simulink model "updatedoldEMS_Gyro_Model"  (R2024a)
settings: Solver=FixedStepAuto  StartTime=0.0  StopTime=360  FixedStep=1/16  RelTol=1e-3
libraries: simulink x1, aerolibnav x1
settings Model: Creator=stevalmontxy  LastModifiedBy=sxyan
settings RTWCC: GPUComputeCapability=3.5

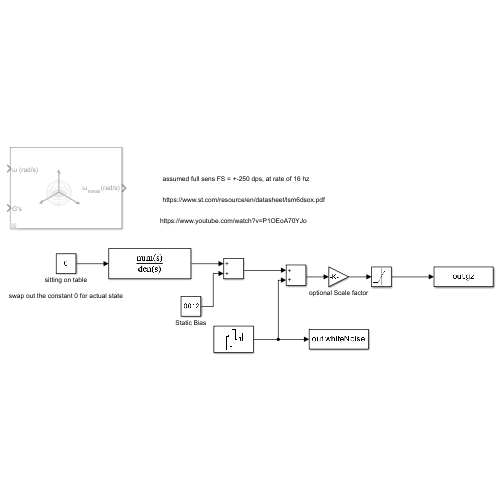
[thumbnail: Simulink's stored preview of the top-level diagram]
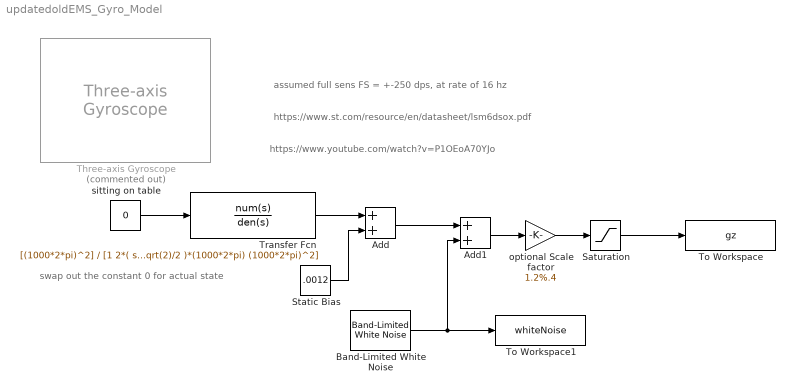
== system updatedoldEMS_Gyro_Model ==
  note: swap out the constant 0 for actual state
  note: https://www.st.com/resource/en/datasheet/lsm6dsox.pdf
  note: assumed full sens FS = +-250 dps, at rate of 16 hz
  note: https://www.youtube.com/watch?v=P1OEoA70YJo
  Add : Sum
  Add1 : Sum
  Band-Limited White Noise : simulink/Sources/Band-Limited White Noise  Cov=".004443^2 %  .0038^2 %"  Ts=1/16  seed=[23341]
  Saturation : Saturate  UpperLimit=2^15  LowerLimit=-2^15
  Static Bias : Constant  Value=.0012
  Three-axis Gyroscope : aerolibnav/Three-axis Gyroscope  Commented=on  dtype_g=on  w_g=190  z_g=0.707  g_sf_cc=[1 0 0; 0 1 0; 0 0 1]  g_bias=[0 0 0]  g_sen=[0 0 0]  g_Ts=0  g_rand=on  g_seeds=[23093 23094 23095]  g_pow=[0.0001 0.0001 0.0001]  g_sat="[-inf  -inf  -inf  inf inf inf]"
  To Workspace : ToWorkspace  VariableName=gz  SampleTime=-1
  To Workspace1 : ToWorkspace  VariableName=whiteNoise  SampleTime=-1
  Transfer Fcn : TransferFcn  Numerator=[(1000*2*pi)^2]  Denominator=[1 2*( sqrt(2)/2 )*(1000*2*pi) (1000*2*pi)^2]
  optional Scale factor : Gain  Gain=1.2%.4
  sitting on table : Constant  Value=0
  wires:
  Static Bias/1 -> Add/2
  Add/1 -> Add1/1
  Add1/1 -> optional Scale factor/1
  Saturation/1 -> To Workspace/1
  optional Scale factor/1 -> Saturation/1
  Transfer Fcn/1 -> Add/1
  sitting on table/1 -> Transfer Fcn/1
  Band-Limited White Noise/1 -> Add1/2, To Workspace1/1
